simulink model "observer_1"  (R2017b)
settings: Solver=ode45  StartTime=0.0  StopTime=10  RelTol=1e-3  EnableMultiTasking=on
undefined symbols (not defined in the file or in its folder): A, H, HT, k, nt, v
settings Model: Creator=Hamid  LastModifiedBy=Sepideh Khakzad
settings DataIOCC: LimitDataPoints=on  SaveFormat=Array
settings OptimizationCC: ExpressionDepthLimit=2147483647  LifeSpan=inf
settings DebuggingCC: UnderspecifiedInitializationDetection=Classic  MergeDetectMultiDrivingBlocksExec=none  SolverPrmCheckMsg=warning  FcnCallInpInsideContextMsg=warning  StateNameClashWarn=warning  SFUnexpectedBacktrackingDiag=warning  SFNoUnconditionalDefaultTransitionDiag=warning  SFExecutionAtInitializationDiag=none
settings HardwareCC: ProdBitPerPointer=32  ProdBitPerSizeT=32  ProdBitPerPtrDiffT=32  ProdLargestAtomicFloat=None  ProdIntDivRoundTo=Undefined  ProdEndianess=Unspecified  ProdWordSize=32  ProdHWDeviceType=32-bit Generic
settings ModelReferenceCC: PropagateSignalLabelsOutOfModel=off
settings CodeAppCC: StateflowObjectComments=on
settings GRTTargetCC: TargetLangStandard=C89/C90 (ANSI)  GeneratePreprocessorConditionals=Disable all  CombineOutputUpdateFcns=off  GRTInterface=on
settings ConfigComp: CovMetricSettings=dw  CovHtmlReporting=on  CovSaveCumulativeToWorkspaceVar=on  CovSaveSingleToWorkspaceVar=on  CovExternalEMLEnable=off

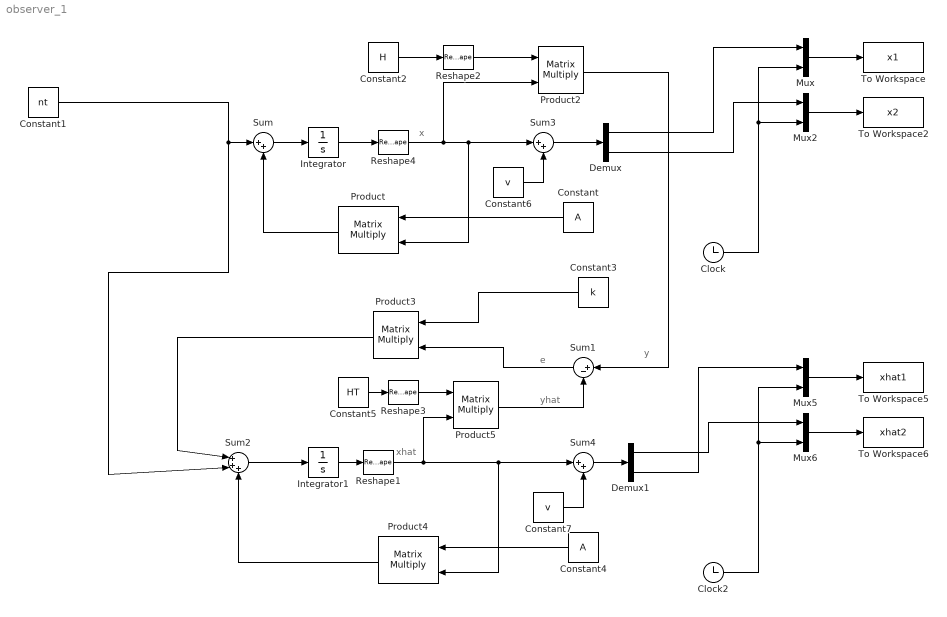
== system observer_1 ==
  note: x
  note: yhat
  note: y
  note: e
  note: xhat
  Clock : Clock
  Clock2 : Clock
  Constant : Constant  Value=A
  Constant1 : Constant  Value=nt
  Constant2 : Constant  Value=H
  Constant3 : Constant  Value=k
  Constant4 : Constant  Value=A
  Constant5 : Constant  Value=HT
  Constant6 : Constant  Value=v
  Constant7 : Constant  Value=v
  Demux : Demux  Outputs=2
  Demux1 : Demux  Outputs=2
  Integrator : Integrator  InitialCondition=[0.15]
  Integrator1 : Integrator
  Mux{,2,5..6} (4 alike) : Mux  Inputs=2
  Product{,2..5} (5 alike) : Product  Multiplication=Matrix(*)  RndMeth=Zero
  Reshape1 : Reshape  OutputDimensionality=Column vector (2-D)
  Reshape2 : Reshape  OutputDimensionality=Row vector (2-D)
  Reshape3 : Reshape  OutputDimensionality=Row vector (2-D)
  Reshape4 : Reshape  OutputDimensionality=Column vector (2-D)  OutputDimensions=[1,2]
  Sum : Sum  Inputs=|++
  Sum1 : Sum  Inputs=|+-
  Sum2 : Sum  Inputs=|+++
  Sum3 : Sum  Inputs=|++
  Sum4 : Sum  Inputs=|++
  To Workspace : ToWorkspace  VariableName=x1  SampleTime=-1
  To Workspace2 : ToWorkspace  VariableName=x2  SampleTime=-1
  To Workspace5 : ToWorkspace  VariableName=xhat1  SampleTime=-1
  To Workspace6 : ToWorkspace  VariableName=xhat2  SampleTime=-1
  wires:
  Product/1 -> Sum/2
  Constant1/1 -> Sum/1, Sum2/2
  Sum/1 -> Integrator/1
  Product2/1 -> Sum1/1
  Sum1/1 -> Product3/2
  Sum2/1 -> Integrator1/1
  Integrator1/1 -> Reshape1/1
  Constant5/1 -> Reshape3/1
  Product5/1 -> Sum1/2
  Product3/1 -> Sum2/1
  Product4/1 -> Sum2/3
  Mux/1 -> To Workspace/1
  Reshape3/1 -> Product5/1
  Mux2/1 -> To Workspace2/1
  Clock/1 -> Mux2/2, Mux/2
  Mux5/1 -> To Workspace5/1
  Mux6/1 -> To Workspace6/1
  Demux1/1 -> Mux6/1
  Demux/1 -> Mux/1
  Demux/2 -> Mux2/1
  Demux1/2 -> Mux5/1
  Clock2/1 -> Mux5/2, Mux6/2
  Constant/1 -> Product/1
  Constant3/1 -> Product3/1
  Constant4/1 -> Product4/1
  Constant2/1 -> Reshape2/1
  Integrator/1 -> Reshape4/1
  Constant6/1 -> Sum3/2
  Sum3/1 -> Demux/1
  Constant7/1 -> Sum4/2
  Reshape1/1 -> Product5/2, Product4/2, Sum4/1
  Sum4/1 -> Demux1/1
  Reshape4/1 -> Product2/2, Sum3/1, Product/2
  Reshape2/1 -> Product2/1
